simulink model "L4_SIM"  (R2018a)
settings: Solver=ode1  StartTime=0.0  StopTime=60  FixedStep=GLB_FIXED_STEP_SIZE_CPV  RelTol=1e-3  EnableMultiTasking=on
undefined symbols (not defined in the file or in its folder): Cf, Chassis, Cr, CYCLE_ACC1_2A__AdaptiveCruiseCtrlMode, CYCLE_ACC1_2A__AdaptiveCruiseCtrlSetSpeed, CYCLE_CCVS1_00__CruiseCtrlSetSpeed, CYCLE_CCVS1_00__WheelBasedVehicleSpeed, CYCLE_EEC1_00__EngSpeed, CYCLE_ETC1_00__TransDrivelineEngaged, CYCLE_ETC2_00__TransActualGearRatio, CYCLE_ETC7_03__TransMode1Indicator, CYCLE_GPS_Latitude, CYCLE_GPS_Longitude, CYCLE_LFE1_00__EngFuelRate, CYCLE_Net_Engine_Percent_Torque, CYCLE_SSI2_03__PitchAngleExRange, CYCLE_TIME, CYCLE_UTM_Origin_X, CYCLE_UTM_Origin_Y, CYCLE_Vehicle_Distance, DiscIntNeverNeededParam, ENUM_J1939_PCC_STATE_T, ENUM_J1939_SWITCH_T, ENUM_STEERING_WHEEL_ANGLE_SENSOR_TYPE_T, GLB_FIXED_STEP_SIZE_CPV, GLB_TRANS_LOSS_TRQ_GEAR_STEP_MPV, GLB_TRANS_LOSS_TRQ_SPD_STEP_MPV, GLB_TRANS_LOSS_TRQ_TABLE_DATA_MPV, GLB_TRANS_LOSS_TRQ_TRQ_STEP_MPV, GLB_VEHICLE_CONFIG_ACCEL_PED_GATEWAY_APV, heading_0, Iz, L4_Controller, lf, lr, position_0, ptc_matlab_lib, STEERCTRL_10ms, SUB_ECU_L4_MABX, SUB_L4_Task_10ms, SUB_L4_Task_10ms_SUB_STEERCTRL, SUB_PLANT_Chassis, Task_10ms, Vx_0
libraries: EmE_MBD_Blockset x81, PTC_MBDS_LIB x71, simulink x38, simulink_extras x1, SUB_L4_Task_10000ms x1, SUB_L4_Task_1000ms x1, SUB_L4_Task_100ms x1, SUB_L4_Task_10ms_SUB_APTC x1, SUB_L4_Task_10ms_SUB_BRKPEDARB x1, SUB_L4_Task_10ms_SUB_FAULT_MANAGER x1, SUB_L4_Task_10ms_SUB_STATE_CONTROL x1, simulink_need_slupdate x1
(part 3 of 6)

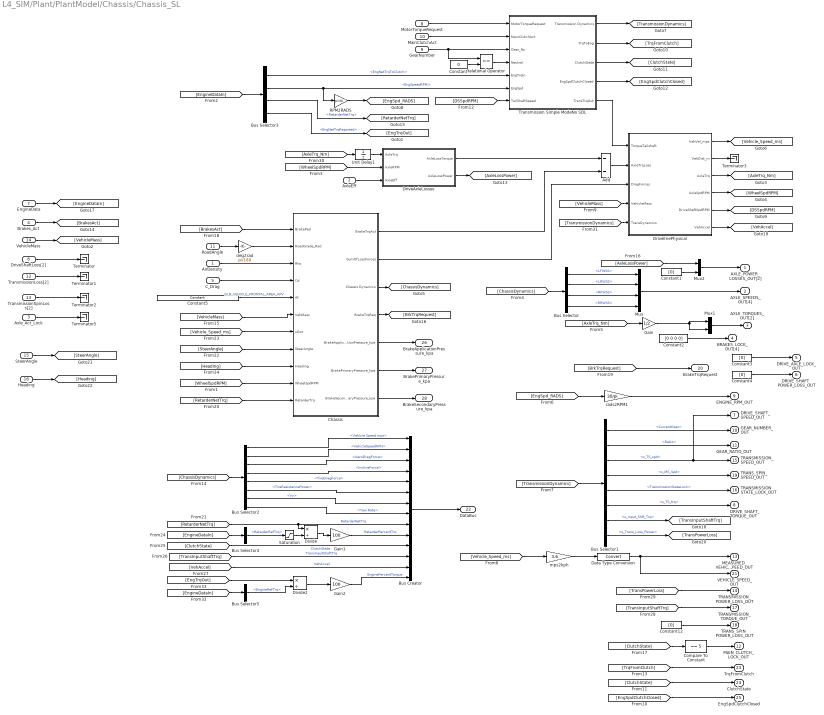
== system L4_SIM/Plant/PlantModel/Chassis/Chassis_SL ==
  AirDensity : Inport
  AxleEff : Inport  Port=2
  Axle_Act_Lock : Inport  Port=3
  Brakes_Act : Inport  Port=4
  C_Drag : Inport  Port=5
  DriveShaftLoss[2] : Inport  Port=6
  EngineData : Inport  Port=7
  MotorTorqueRequest : Inport  Port=8
  GearNumber : Inport  Port=9
  MainClutchAct : Inport  Port=10
  RoadAngle : Inport  Port=11
  TransmissionLoss[2] : Inport  Port=12
  TransmissionSpinLoss[2] : Inport  Port=13
  VehicleMass : Inport  Port=14
  SteerAngle : Inport  Port=15
  Heading : Inport  Port=16
  Add : Sum  Inputs=--
  Bus Creator : BusCreator  Inputs=14
  Bus Selector : BusSelector  OutputSignals=Wheel Speed Sensors.LFWSS,Wheel Speed Sensors.LRWSS,Wheel Speed Sensors.RFWSS,Wheel Speed Sensors.RRWSS
  Bus Selector1 : BusSelector  OutputSignals=Gears_bus.CurrentGear,Gears_bus.Ratio,Gears_bus.s_TS_spd,Gears_bus.s_MS_Spd,MainClutch_bus.TransmissionStateLock,Gears_bus.s_TS_trq,s_Input_Shft_Trq,Gears_bus.s_Trans_Loss_Power
  Bus Selector2 : BusSelector  OutputSignals=Vehicle Speed mps,VehicleSpeedKPH,LongitudnalDynamics.AeroDragForce,LongitudnalDynamics.InclineForce,LongitudnalDynamics.TireDragForce,TireResistancePower,LateralDynamics.Vy,LateralDynamics.Yaw Rate
  Bus Selector3 : BusSelector  OutputSignals=EngNetTrqToClutch,EngSpeedRPM,RetarderNetTrq,EngNetTrqReported
  Bus Selector4 : BusSelector  OutputSignals=RetarderRefTrq
  Bus Selector5 : BusSelector  OutputSignals=EngineRefTrq
  Chassis : Subsystem
  Compare To Constant : simulink/Logic and Bit Operations/Compare To Constant  relop===  const=5  OutDataTypeStr=boolean
  Constant : Constant  Value=0
  Constant{1,3..4,12} (4 alike) : Constant  Value=[0]
  Constant2 : Constant  Value=[0 0 0 0]
  Constant5 : PTC_MBDS_LIB/Extras/Sources/Constant  Value2=GLB_VEHICLE_FRONTAL_AREA_APV  PTC_MBDS_BlockVersion=5.41  PTC_BlockType=PTC_MBDS_Constant
      settings: SourceProductName=PACCAR Technical Center MBDS Library
      settings: AttributesFormatString=|
      | Value: 10.38
      | Unit: 'm^2'
  Data Type Conversion : DataTypeConversion  SaturateOnIntegerOverflow=on
  Divide : Product  Inputs=*/
  Divide2 : Product  Inputs=*/
  DriveAxleLosses : Subsystem
  DrivelInePhysical : Subsystem
  Gain : Gain  Gain=1/2
  Gain1 : Gain  Gain=100
  Gain2 : Gain  Gain=100
  Mux : Mux
  Mux1 : Mux  Inputs=2
  Mux2 : Mux  Inputs=2
  RPM2RADS : Gain  Gain=pi/30
  Relational Operator : RelationalOperator  Operator===  OutDataTypeStr=boolean  RndMeth=Nearest
  Saturation : Saturate  UpperLimit=inf  LowerLimit=1
  Terminator{,1..3,5} (5 alike) : Terminator
      Terminator3 settings: InitFcn=|
      | try
      |    MBDS_BlockCallback('Update', gcb);
      | end
  Transmission Simple ModeNo SDL : Subsystem
  Unit Delay1 : UnitDelay  SampleTime=-1
  deg2rad : Gain  Gain=pi/180
  mps2kph : Gain  Gain=3.6
  rads2RPM1 : Gain  Gain=30/pi
  AXLE_POWER_LOSSES_OUT[2] : Outport
  AXLE_SPEEDS_OUT[4] : Outport  Port=2
  AXLE_TORQUES_OUT[2] : Outport  Port=3
  BRAKES_LOCK_OUT[4] : Outport  Port=4
  DRIVE_AXLE_LOCK_OUT : Outport  Port=5
  DRIVE_SHAFT_POWER_LOSS_OUT : Outport  Port=6
  DRIVE_SHAFT_SPEED_OUT : Outport  Port=7
  DRIVE_SHAFT_TORQUE_OUT : Outport  Port=8
  ENGINE_RPM_OUT : Outport  Port=9
  GEAR_NUMBER_OUT : Outport  Port=10
  GEAR_RATIO_OUT : Outport  Port=11
  MAIN_CLUTCH_LOCK_OUT : Outport  Port=12
  MEASURED_VEHICLE_SPEED_OUT : Outport  Port=13
  TRANSMISSION_POWER_LOSS_OUT : Outport  Port=14
  TRANSMISSION_SPEED_OUT : Outport  Port=15
  TRANSMISSION_STATE_LOCK_OUT : Outport  Port=16
  TRANSMISSION_TORQUE_OUT : Outport  Port=17
  TRANS_SPIN_POWER_LOSS_OUT : Outport  Port=18
  TRANS_SPIN_SPEED_OUT : Outport  Port=19
  BrakeTrqRequest : Outport  Port=20
  VEHICLE_SPEED_OUT : Outport  Port=21
  DataBus : Outport  Port=22
  TrqFromClutch : Outport  Port=23
  ClutchState : Outport  Port=24
  EngSpdClutchClosed : Outport  Port=25
  BrakeApplicationPressure_kpa : Outport  Port=26
  BrakePrimaryPressure_kpa : Outport  Port=27
  BrakeSecondaryPressure_kpa : Outport  Port=28
  wires:
  DrivelInePhysical/1(VehVel_mps) -> [Vehicle_Speed_ms]
  Heading/1 -> [Heading]
  [Heading] -> Chassis/9(Heading)
  Bus Selector2/8 -> Bus Creator/8  "<Yaw Rate>"
  Bus Selector2/7 -> Bus Creator/7  "<Vy>"
  [SteerAngle] -> Chassis/8(SteerAngle)
  SteerAngle/1 -> [SteerAngle]
  Chassis/7(BrakeSecondaryPressure_kpa) -> BrakeSecondaryPressure_kpa/1
  Chassis/6(BrakePrimaryPressure_kpa) -> BrakePrimaryPressure_kpa/1
  Chassis/5(BrakeApplicationPressure_kpa) -> BrakeApplicationPressure_kpa/1
  Gain2/1 -> Bus Creator/14  "EnginePercentTorque"
  Divide2/1 -> Gain2/1
  [EngTrqOut] -> Divide2/1
  Bus Selector5/1 -> Divide2/2  "<EngineRefTrq>"
  [EngineDataIn] -> Bus Selector5/1
  Bus Selector/4 -> Mux/4  "<RRWSS>"
  Bus Selector/3 -> Mux/3  "<RFWSS>"
  Bus Selector/2 -> Mux/2  "<LRWSS>"
  Bus Selector/1 -> Mux/1  "<LFWSS>"
  Data Type Conversion/1 -> MEASURED_VEHICLE_SPEED_OUT/1, VEHICLE_SPEED_OUT/1
  Unit Delay1/1 -> DriveAxleLosses/1(AxleTrq)
  [TransmissionDynamics] -> DrivelInePhysical/5(TransDynamics)
  Bus Selector1/8 -> [TransPowerLoss]  "<s_Trans_Loss_Power>"
  Bus Selector2/5 -> Bus Creator/5  "<TireDragForce>"
  Saturation/1 -> Divide/2
  [VehAccel] -> Bus Creator/13  "VehAccel"
  DrivelInePhysical/6(VehAccel) -> [VehAccel]
  [TransInputShaftTrq] -> Bus Creator/12  "TransInputShaftTrq"
  Bus Selector1/7 -> [TransInputShaftTrq]  "<s_Input_Shft_Trq>"
  [ClutchState] -> Bus Creator/11  "ClutchState"
  Gain1/1 -> Bus Creator/10  "RetarderPercentTrq"
  Divide/1 -> Gain1/1
  Bus Selector4/1 -> Saturation/1  "<RetarderRefTrq>"
  [EngineDataIn] -> Bus Selector4/1
  EngineData/1 -> [EngineDataIn]
  Bus Selector2/6 -> Bus Creator/6  "<TireResistancePower>"
  Bus Selector2/4 -> Bus Creator/4  "<InclineForce>"
  Bus Selector2/3 -> Bus Creator/3  "<AeroDragForce>"
  Bus Selector2/2 -> Bus Creator/2  "<VehicleSpeedKPH>"
  Bus Selector2/1 -> Bus Creator/1  "<Vehicle Speed mps>"
  [RetarderNetTrq] -> Divide/1, Bus Creator/9  "RetarderNetTrq"
  Bus Creator/1 -> DataBus/1
  [RetarderNetTrq] -> Chassis/11(RetarderTrq)
  Chassis/4(BrakeTrqReq) -> [BrkTrqRequest]
  Bus Selector3/4 -> [EngTrqOut]  "<EngNetTrqReported>"
  Brakes_Act/1 -> [BrakesAct]
  [ClutchState] -> Compare To Constant/1
  Constant1/1 -> Mux2/2
  [AxleLossPower] -> Mux2/1
  DriveAxleLosses/2(AxleLossPower) -> [AxleLossPower]
  [VehicleMass] -> Chassis/6(VehMass)
  [ChassisDynamics] -> Bus Selector2/1
  RPM2RADS/1 -> [EngSpd_RADS]
  Transmission Simple ModeNo SDL/5(TransTrqOut) -> DrivelInePhysical/1(TorqueTailshaft)
  [EngSpdClutchClosed] -> EngSpdClutchClosed/1
  Transmission Simple ModeNo SDL/4(EngSpdClutchClosed) -> [EngSpdClutchClosed]
  Bus Selector3/1 -> Transmission Simple ModeNo SDL/5(EngTrqIn)  "<EngNetTrqToClutch>"
  [TrqFromClutch] -> TrqFromClutch/1
  [ClutchState] -> ClutchState/1
  Transmission Simple ModeNo SDL/3(ClutchState) -> [ClutchState]
  Transmission Simple ModeNo SDL/2(TrqToEng) -> [TrqFromClutch]
  [DSSpdRPM] -> Transmission Simple ModeNo SDL/7(TailShaftSpeed)
  DrivelInePhysical/5(DriveShaftSpdRPM) -> [DSSpdRPM]
  [VehicleMass] -> DrivelInePhysical/4(VehicleMass)
  VehicleMass/1 -> [VehicleMass]
  [WheelSpdRPM] -> Chassis/10(WheelSpdRPM)
  DrivelInePhysical/4(AxleSpdRPM) -> [WheelSpdRPM]
  Bus Selector1/3 -> DRIVE_SHAFT_SPEED_OUT/1, TRANSMISSION_SPEED_OUT/1  "<s_TS_spd>"
  [BrkTrqRequest] -> BrakeTrqRequest/1
  Bus Selector1/4 -> TRANS_SPIN_SPEED_OUT/1  "<s_MS_Spd>"
  Constant12/1 -> TRANS_SPIN_POWER_LOSS_OUT/1
  [TransInputShaftTrq] -> TRANSMISSION_TORQUE_OUT/1
  Bus Selector1/5 -> TRANSMISSION_STATE_LOCK_OUT/1  "<TransmissionStateLock>"
  [TransPowerLoss] -> TRANSMISSION_POWER_LOSS_OUT/1
  mps2kph/1 -> Data Type Conversion/1
  [Vehicle_Speed_ms] -> mps2kph/1
  Compare To Constant/1 -> MAIN_CLUTCH_LOCK_OUT/1
  Bus Selector1/2 -> GEAR_RATIO_OUT/1  "<Ratio>"
  Bus Selector1/1 -> GEAR_NUMBER_OUT/1  "<CurrentGear>"
  [TransmissionDynamics] -> Bus Selector1/1
  rads2RPM1/1 -> ENGINE_RPM_OUT/1
  [EngSpd_RADS] -> rads2RPM1/1
  Gain/1 -> Mux1/1, Mux1/2
  [AxleTrq_Nm] -> Gain/1
  Bus Selector1/6 -> DRIVE_SHAFT_TORQUE_OUT/1  "<s_TS_trq>"
  Constant4/1 -> DRIVE_SHAFT_POWER_LOSS_OUT/1
  Constant3/1 -> DRIVE_AXLE_LOCK_OUT/1
  Mux1/1 -> AXLE_TORQUES_OUT[2]/1
  Mux/1 -> AXLE_SPEEDS_OUT[4]/1
  Constant2/1 -> BRAKES_LOCK_OUT[4]/1
  Mux2/1 -> AXLE_POWER_LOSSES_OUT[2]/1
  [ChassisDynamics] -> Bus Selector/1
  Transmission Simple ModeNo SDL/1(Transmission Dynamics) -> [TransmissionDynamics]
  Chassis/3(Chassis Dynamics) -> [ChassisDynamics]
  Axle_Act_Lock/1 -> Terminator5/1
  TransmissionSpinLoss[2]/1 -> Terminator2/1
  TransmissionLoss[2]/1 -> Terminator1/1
  DriveShaftLoss[2]/1 -> Terminator/1
  [WheelSpdRPM] -> DriveAxleLosses/2(AxleRPM)
  AxleEff/1 -> DriveAxleLosses/3(AxleEff)
  [AxleTrq_Nm] -> Unit Delay1/1
  DrivelInePhysical/3(AxleTrq) -> [AxleTrq_Nm]
  Add/1 -> DrivelInePhysical/2(AxleTrqLoss)
  Chassis/1(BrakeTrqAct) -> Add/2
  DriveAxleLosses/1(AxleLossTorque) -> Add/1
  DrivelInePhysical/2(VehDist_m) -> Terminator3/1
  [Vehicle_Speed_ms] -> Chassis/7(xDot)
  [BrakesAct] -> Chassis/1(BrakePed)
  Chassis/2(SumOfLossForces) -> DrivelInePhysical/3(DragForces)
  Constant/1 -> Relational Operator/2
  Relational Operator/1 -> Transmission Simple ModeNo SDL/4(Neutral)
  GearNumber/1 -> Transmission Simple ModeNo SDL/3(Gear_No), Relational Operator/1
  MainClutchAct/1 -> Transmission Simple ModeNo SDL/2(MainClutchAct)
  deg2rad/1 -> Chassis/2(RoadGrade_Rad)
  RoadAngle/1 -> deg2rad/1
  Constant5/1 -> Chassis/5(Af)  "GLB_VEHICLE_FRONTAL_AREA_APV"
  C_Drag/1 -> Chassis/4(Cd)
  AirDensity/1 -> Chassis/3(Rho)
  [EngineDataIn] -> Bus Selector3/1
  Bus Selector3/2 -> RPM2RADS/1, Transmission Simple ModeNo SDL/6(EngSpd)  "<EngSpeedRPM>"
  Bus Selector3/3 -> [RetarderNetTrq]  "<RetarderNetTrq>"
  MotorTorqueRequest/1 -> Transmission Simple ModeNo SDL/1(MotorTorqueRequest)

== system L4_SIM/Controllers/Operator/Subsystem/SpdControlBrake/SpdControlBrake ==
  VehSpdTarget : Inport
  VehSpdAct : Inport  Port=2
  Kp : Inport  Port=3
  Ti : Inport  Port=4
  Td : Inport  Port=5
  Reset : Inport  Port=6
  Constant : Constant  Value=0
  Constant1 : Constant  Value=0
  Constant2 : Constant  Value=-1
  Constant3 : Constant
  Constant4 : PTC_MBDS_LIB/Extras/Sources/Constant  Value2=GLB_FIXED_STEP_SIZE_CPV  PTC_MBDS_BlockVersion=5.41  PTC_BlockType=PTC_MBDS_Constant
      settings: SourceProductName=PACCAR Technical Center MBDS Library
      settings: AttributesFormatString=|
      | Value: 0.01
      | Unit: 's'
  Constant7 : Constant
  Constant8 : Constant  Value=0
  Gain : Gain  Gain=-1
  Mux : Mux
  PID : Subsystem
  Relational Operator : RelationalOperator  OutDataTypeStr=boolean  RndMeth=Nearest
  Relational Operator1 : RelationalOperator  Operator=<=  OutDataTypeStr=boolean  RndMeth=Nearest
  Saturation Dynamic : simulink/Discontinuities/Saturation Dynamic  RequirementInfo={} %GIDa_73e9c469_c4a7_47ae_bea8_3c2217de47e7  OutMin=[]  OutMax=[]  OutDataTypeStr=Inherit: Same as second input  OutDataType=sfix(16)  OutScaling=2^-10  DoSatur=off
  Switch : Switch  Criteria=u2 ~= 0
  Switch1 : Switch  Criteria=u2 ~= 0
  Terminator : Terminator
  Unit Delay : UnitDelay  SampleTime=-1
  BrakeComGov(0-1) : Outport
  wires:
  Reset/1 -> PID/2(Reset_Integral)
  Saturation Dynamic/1 -> BrakeComGov(0-1)/1
  Gain/1 -> Saturation Dynamic/2, Unit Delay/1
  Td/1 -> PID/7(Td)
  Unit Delay/1 -> Relational Operator1/1, Relational Operator/1
  Constant8/1 -> Saturation Dynamic/3, Relational Operator1/2
  Constant7/1 -> Saturation Dynamic/1, Relational Operator/2
  Relational Operator/1 -> Switch/2
  Constant3/1 -> Switch/1
  Switch1/1 -> Switch/3
  Constant2/1 -> Switch1/1
  Constant/1 -> Switch1/3
  Relational Operator1/1 -> Switch1/2
  Switch/1 -> PID/9(Sat_state)
  PID/4(D_Out1) -> Mux/4
  PID/3(I_Out) -> Mux/3
  PID/2(P_Out) -> Mux/2
  Mux/1 -> Terminator/1
  Constant1/1 -> PID/1(Init)
  Kp/1 -> PID/5(K)
  Ti/1 -> PID/6(Ti)
  Constant4/1 -> PID/8(Ts)  "GLB_FIXED_STEP_SIZE_CPV"
  VehSpdTarget/1 -> PID/3(SP)
  VehSpdAct/1 -> PID/4(FB)
  PID/1(Out1) -> Gain/1, Mux/1

== system L4_SIM/Controllers/Operator/Subsystem/SpdControlTraction/SpdControlTraction ==
  VehSpdTarget : Inport
  VehSpdAct : Inport  Port=2
  Kp : Inport  Port=3
  Ti : Inport  Port=4
  Td : Inport  Port=5
  Reset : Inport  Port=6
  Constant : Constant  Value=0
  Constant1 : Constant  Value=0
  Constant2 : Constant  Value=-1
  Constant3 : Constant
  Constant4 : PTC_MBDS_LIB/Extras/Sources/Constant  Value2=GLB_FIXED_STEP_SIZE_CPV  PTC_MBDS_BlockVersion=5.41  PTC_BlockType=PTC_MBDS_Constant
      settings: SourceProductName=PACCAR Technical Center MBDS Library
      settings: AttributesFormatString=|
      | Value: 0.01
      | Unit: 's'
  Constant7 : Constant
  Constant8 : Constant  Value=0
  Mux : Mux
  PID : Subsystem
  Relational Operator : RelationalOperator  OutDataTypeStr=boolean  RndMeth=Nearest
  Relational Operator1 : RelationalOperator  Operator=<=  OutDataTypeStr=boolean  RndMeth=Nearest
  Saturation : Saturate  UpperLimit=1  LowerLimit=0
  Switch : Switch  Criteria=u2 ~= 0
  Switch1 : Switch  Criteria=u2 ~= 0
  Terminator : Terminator
  Unit Delay : UnitDelay  SampleTime=-1
  PedalComGov(0-1) : Outport
  wires:
  Switch/1 -> PID/9(Sat_state)
  Unit Delay/1 -> Relational Operator1/1, Relational Operator/1
  Constant8/1 -> Relational Operator1/2
  Constant7/1 -> Relational Operator/2
  Relational Operator/1 -> Switch/2
  Constant3/1 -> Switch/1
  Switch1/1 -> Switch/3
  Constant2/1 -> Switch1/1
  Constant/1 -> Switch1/3
  Relational Operator1/1 -> Switch1/2
  PID/4(D_Out1) -> Mux/4
  PID/3(I_Out) -> Mux/3
  PID/2(P_Out) -> Mux/2
  Mux/1 -> Terminator/1
  Constant4/1 -> PID/8(Ts)  "GLB_FIXED_STEP_SIZE_CPV"
  PID/1(Out1) -> Unit Delay/1, Saturation/1, Mux/1
  Saturation/1 -> PedalComGov(0-1)/1
  VehSpdTarget/1 -> PID/3(SP)
  VehSpdAct/1 -> PID/4(FB)
  Kp/1 -> PID/5(K)
  Ti/1 -> PID/6(Ti)
  Td/1 -> PID/7(Td)
  Constant1/1 -> PID/1(Init)
  Reset/1 -> PID/2(Reset_Integral)

== system L4_SIM/Controllers/Virtual_Controllers/Interface_Abstraction/CAN/ACC1 ==
  SPN1586_SpeedOfForwardVehicle : Inport
  SPN1587_DistanceToForwardVehicle : Inport  Port=2
  SPN1588_AdaptiveCruiseControlSetSpeed : Inport  Port=3
  SPN1590_AdaptiveCruiseControlMode : Inport  Port=4
  SPN1589_AdaptiveCruiseControlSetDistMode : Inport  Port=5
  SPN1591_RoadCurvature : Inport  Port=6
  SPN1798_ACC_TargetDetected : Inport  Port=7
  SPN1797_ACC_SystemShutoffWarning : Inport  Port=8
  SPN1796_ACC_DistanceAlertSignal : Inport  Port=9
  SPN5022_ForwardCollisionWarning : Inport  Port=10
  Bus Creator2 : BusCreator  Inputs=10
  ACC1 : Outport
  wires:
  SPN1586_SpeedOfForwardVehicle/1 -> Bus Creator2/1  "SPN1586_SpeedOfForwardVehicle"
  Bus Creator2/1 -> ACC1/1  "ACC1"
  SPN1587_DistanceToForwardVehicle/1 -> Bus Creator2/2  "SPN1587_DistanceToForwardVehicle"
  SPN1588_AdaptiveCruiseControlSetSpeed/1 -> Bus Creator2/3  "SPN1588_AdaptiveCruiseControlSetSpeed"
  SPN1590_AdaptiveCruiseControlMode/1 -> Bus Creator2/4  "SPN1590_AdaptiveCruiseControlMode"
  SPN1797_ACC_SystemShutoffWarning/1 -> Bus Creator2/8  "SPN1797_ACC_SystemShutoffWarning"
  SPN1798_ACC_TargetDetected/1 -> Bus Creator2/7  "SPN1798_ACC_TargetDetected"
  SPN1591_RoadCurvature/1 -> Bus Creator2/6  "SPN1591_RoadCurvature"
  SPN1589_AdaptiveCruiseControlSetDistMode/1 -> Bus Creator2/5  "SPN1589_AdaptiveCruiseControlSetDistMode"
  SPN1796_ACC_DistanceAlertSignal/1 -> Bus Creator2/9  "SPN1796_ACC_DistanceAlertSignal"
  SPN5022_ForwardCollisionWarning/1 -> Bus Creator2/10  "SPN5022_ForwardCollisionWarning"

== system L4_SIM/Controllers/Virtual_Controllers/Interface_Abstraction/CAN/AMB ==
  SPN108_BarometricPressure : Inport
  SPN171_AmbientAirTemperature : Inport  Port=2
  SPN170_CabInteriorTemperature : Inport  Port=3
  Bus Creator2 : BusCreator  Inputs=3
  AMB : Outport
  wires:
  Bus Creator2/1 -> AMB/1
  SPN108_BarometricPressure/1 -> Bus Creator2/1  "SPN108_BarometricPressure"
  SPN171_AmbientAirTemperature/1 -> Bus Creator2/2  "SPN171_AmbientAirTemperature"
  SPN170_CabInteriorTemperature/1 -> Bus Creator2/3  "SPN170_CabInteriorTemperature"

== system L4_SIM/Controllers/Virtual_Controllers/Interface_Abstraction/CAN/BrakeSwitch ==
  In : Inport
  Compare To Constant : simulink/Logic and Bit Operations/Compare To Constant  relop=>=  const=0.05  OutDataTypeStr=boolean
  Out : Outport
  wires:
  In/1 -> Compare To Constant/1
  Compare To Constant/1 -> Out/1

== system L4_SIM/Controllers/Virtual_Controllers/Interface_Abstraction/CAN/CC ==
  CCSetSpd : Inport
  Constant : Constant  Value=20
  Constant1 : Constant
  Constant2 : Constant  Value=0
  Relational Operator : RelationalOperator  Operator=>  OutDataTypeStr=boolean  RndMeth=Nearest
  Switch : Switch  Criteria=u2 ~= 0
  CruiseActive : Outport
  CruiseState : Outport  Port=2
  wires:
  Relational Operator/1 -> Switch/2, CruiseActive/1
  Constant/1 -> Relational Operator/2
  CCSetSpd/1 -> Relational Operator/1
  Switch/1 -> CruiseState/1
  Constant1/1 -> Switch/1
  Constant2/1 -> Switch/3

== system L4_SIM/Controllers/Virtual_Controllers/Interface_Abstraction/CAN/CCVS1 ==
  SPN84_WheelBasedVehicleSpeed : Inport
  SPN597_BrakeSwitch : Inport  Port=2
  SPN86_CruiseControlSetSpeed : Inport  Port=3
  SPN595_CruiseControlActive : Inport  Port=4
  SPN527_CruiseControlState : Inport  Port=5
  Bus Creator2 : BusCreator  Inputs=5
  CCVS1 : Outport
  wires:
  SPN84_WheelBasedVehicleSpeed/1 -> Bus Creator2/1
  Bus Creator2/1 -> CCVS1/1
  SPN597_BrakeSwitch/1 -> Bus Creator2/2
  SPN86_CruiseControlSetSpeed/1 -> Bus Creator2/3
  SPN595_CruiseControlActive/1 -> Bus Creator2/4
  SPN527_CruiseControlState/1 -> Bus Creator2/5

== system L4_SIM/Controllers/Virtual_Controllers/Interface_Abstraction/CAN/CCVS3 ==
  SPN7319_CruiseControlSpeed : Inport
  Bus Creator2 : BusCreator  Inputs=1
  CCVS3 : Outport
  wires:
  Bus Creator2/1 -> CCVS3/1
  SPN7319_CruiseControlSpeed/1 -> Bus Creator2/1

== system L4_SIM/Controllers/Virtual_Controllers/Interface_Abstraction/CAN/CVW ==
  SPN1760_GrossCombinationVehicleWeight : Inport
  Bus Creator2 : BusCreator  Inputs=1
  CVW : Outport
  wires:
  Bus Creator2/1 -> CVW/1
  SPN1760_GrossCombinationVehicleWeight/1 -> Bus Creator2/1

== system L4_SIM/Controllers/Virtual_Controllers/Interface_Abstraction/CAN/EBC1 ==
  SPN521_BrakePedalPosition : Inport
  Bus Creator2 : BusCreator  Inputs=2
  Constant : Constant  Value=0
  Relational Operator : RelationalOperator  Operator=>  OutDataTypeStr=boolean  RndMeth=Simplest
  EBC1 : Outport
  wires:
  SPN521_BrakePedalPosition/1 -> Relational Operator/1, Bus Creator2/1
  Bus Creator2/1 -> EBC1/1
  Constant/1 -> Relational Operator/2
  Relational Operator/1 -> Bus Creator2/2  "SPN1121_EBS_BrakeSwitch"

== system L4_SIM/Controllers/Virtual_Controllers/Interface_Abstraction/CAN/EBC2 ==
  SPN904_FrontAxleSpd : Inport  Unit=km/h
  Bus Creator2 : BusCreator  Inputs=1
  EBC2 : Outport
  wires:
  Bus Creator2/1 -> EBC2/1
  SPN904_FrontAxleSpd/1 -> Bus Creator2/1  "SPN904_FrontAxleSpd"

== system L4_SIM/Controllers/Virtual_Controllers/Interface_Abstraction/CAN/EC1 ==
  SPN544_EngineReferenceTrq : Inport
  Bus Creator2 : BusCreator  Inputs=1
  EC1 : Outport
  wires:
  SPN544_EngineReferenceTrq/1 -> Bus Creator2/1  "SPN544_EngineReferenceTrq"
  Bus Creator2/1 -> EC1/1

== system L4_SIM/Controllers/Virtual_Controllers/Interface_Abstraction/CAN/EEC1 ==
  SPN512_DriverDemandPercTorque : Inport
  SPN513_ActualEngPercTorque : Inport  Port=2
  SPN4154_ActualEngPercTorqueFractional : Inport  Port=3
  SPN190_EngineSpeed : Inport  Port=4
  Bus Creator : BusCreator  Inputs=4
  EEC1 : Outport
  wires:
  Bus Creator/1 -> EEC1/1
  SPN190_EngineSpeed/1 -> Bus Creator/4
  SPN4154_ActualEngPercTorqueFractional/1 -> Bus Creator/3
  SPN513_ActualEngPercTorque/1 -> Bus Creator/2
  SPN512_DriverDemandPercTorque/1 -> Bus Creator/1

== system L4_SIM/Controllers/Virtual_Controllers/Interface_Abstraction/CAN/EEC2 ==
  SPN91_AccelPedalPosition1 : Inport
  Bus Creator2 : BusCreator  Inputs=1
  EEC2 : Outport
  wires:
  Bus Creator2/1 -> EEC2/1
  SPN91_AccelPedalPosition1/1 -> Bus Creator2/1

== system L4_SIM/Controllers/Virtual_Controllers/Interface_Abstraction/CAN/EEC3 ==
  SPN514_NominalFrictionPercTorque : Inport
  SPN2978_EstimatedEngineParasiticLossesPercTrq : Inport  Port=2
  Bus Creator2 : BusCreator  Inputs=2
  EEC3 : Outport
  wires:
  Bus Creator2/1 -> EEC3/1
  SPN514_NominalFrictionPercTorque/1 -> Bus Creator2/1  "SPN514_NominalFrictionPercTorque"
  SPN2978_EstimatedEngineParasiticLossesPercTrq/1 -> Bus Creator2/2  "SPN2978_EstimatedEngineParasiticLossesPercTrq"

== system L4_SIM/Controllers/Virtual_Controllers/Interface_Abstraction/CAN/ERC1 ==
  SPN520_ActualRetarderPercentTorque : Inport
  SPN1715_DriverDemandRetarderPercentTorque : Inport  Port=2
  Bus Creator2 : BusCreator  Inputs=2
  ERC1 : Outport
  wires:
  SPN520_ActualRetarderPercentTorque/1 -> Bus Creator2/1
  Bus Creator2/1 -> ERC1/1
  SPN1715_DriverDemandRetarderPercentTorque/1 -> Bus Creator2/2

== system L4_SIM/Controllers/Virtual_Controllers/Interface_Abstraction/CAN/ETC1 ==
  SPN560_TransDrivelineEngaged : Inport
  Bus Creator2 : BusCreator  Inputs=1
  ETC1 : Outport
  wires:
  Bus Creator2/1 -> ETC1/1  "ETC1"
  SPN560_TransDrivelineEngaged/1 -> Bus Creator2/1

== system L4_SIM/Controllers/Virtual_Controllers/Interface_Abstraction/CAN/ETC2 ==
  SPN524_TransSelectedGear : Inport
  SPN526_TransActualGearRatio : Inport  Port=2
  SPN523_TransCurrentGear : Inport  Port=3
  Bus Creator1 : BusCreator  Inputs=3
  ETC2 : Outport
  wires:
  Bus Creator1/1 -> ETC2/1
  SPN526_TransActualGearRatio/1 -> Bus Creator1/2
  SPN523_TransCurrentGear/1 -> Bus Creator1/3
  SPN524_TransSelectedGear/1 -> Bus Creator1/1

== system L4_SIM/Controllers/Virtual_Controllers/Interface_Abstraction/CAN/GNSSSDOP ==
  SID : Inport
  SetMode : Inport  Port=2
  OpMode : Inport  Port=3
  HDOP : Inport  Port=4
  VDOP : Inport  Port=5
  TDOP : Inport  Port=6
  Bus Creator2 : BusCreator  Inputs=6
  GNSSDOP : Outport
  wires:
  Bus Creator2/1 -> GNSSDOP/1
  SID/1 -> Bus Creator2/1  "SID"
  SetMode/1 -> Bus Creator2/2  "SetMode"
  OpMode/1 -> Bus Creator2/3  "OpMode"
  HDOP/1 -> Bus Creator2/4  "HDOP"
  VDOP/1 -> Bus Creator2/5  "VDOP"
  TDOP/1 -> Bus Creator2/6  "TDOP"

== system L4_SIM/Controllers/Virtual_Controllers/Interface_Abstraction/CAN/HRW ==
  SPN1592_FrontAxleLeftWheelSpeed : Inport  Unit=km/h
  SPN1593_FrontAxleRightWheelSpeed : Inport  Port=2  Unit=km/h
  SPN1594_RearAxleLeftWheelSpeed : Inport  Port=3  Unit=km/h
  SPN1595_RearAxleRightWheelSpeed : Inport  Port=4  Unit=km/h
  Bus Creator2 : BusCreator  Inputs=4
  HRW_0B : Outport
  wires:
  SPN1592_FrontAxleLeftWheelSpeed/1 -> Bus Creator2/1  "SPN1592_FrontAxleLeftWheelSpeed"
  Bus Creator2/1 -> HRW_0B/1
  SPN1593_FrontAxleRightWheelSpeed/1 -> Bus Creator2/2  "SPN1593_FrontAxleRightWheelSpeed"
  SPN1594_RearAxleLeftWheelSpeed/1 -> Bus Creator2/3  "SPN1594_RearAxleLeftWheelSpeed"
  SPN1595_RearAxleRightWheelSpeed/1 -> Bus Creator2/4  "SPN1595_RearAxleRightWheelSpeed"

== system L4_SIM/Controllers/Virtual_Controllers/Interface_Abstraction/CAN/PCC1 ==
  SPN7316_PCCSetSpeedOffset : Inport
  SPN7317_PCCState : Inport  Port=2
  SPN7430_PCCDrivelineDisengageInhibit : Inport  Port=3
  Bus Creator2 : BusCreator  Inputs=3
  PCC1 : Outport
  wires:
  Bus Creator2/1 -> PCC1/1
  SPN7316_PCCSetSpeedOffset/1 -> Bus Creator2/1
  SPN7317_PCCState/1 -> Bus Creator2/2
  SPN7430_PCCDrivelineDisengageInhibit/1 -> Bus Creator2/3

== system L4_SIM/Controllers/Virtual_Controllers/Interface_Abstraction/CAN/PosRapidUpdate ==
  Latitude : Inport
  Longitude : Inport  Port=2
  Bus Creator2 : BusCreator  Inputs=2
  PosRapidUpdate : Outport
  wires:
  Longitude/1 -> Bus Creator2/2  "Longitude"
  Latitude/1 -> Bus Creator2/1  "Latitude"
  Bus Creator2/1 -> PosRapidUpdate/1

== system L4_SIM/Controllers/Virtual_Controllers/Interface_Abstraction/CAN/SSI2 ==
  SPN4976_PitchAngleExtendedRange : Inport
  Bus Creator2 : BusCreator  Inputs=1
  SSI2 : Outport
  wires:
  SPN4976_PitchAngleExtendedRange/1 -> Bus Creator2/1
  Bus Creator2/1 -> SSI2/1  "ETC1"

== system L4_SIM/Controllers/Virtual_Controllers/Interface_Abstraction/CAN/TransDrivelineEngaged ==
  In1 : Inport
  Constant : PTC_MBDS_LIB/Extras/Sources/Constant  Value2=ENUM_J1939_SWITCH_T.ON  PTC_MBDS_BlockVersion=5.41  PTC_BlockType=PTC_MBDS_Constant
      settings: SourceProductName=PACCAR Technical Center MBDS Library
  Constant1 : PTC_MBDS_LIB/Extras/Sources/Constant  Value2=ENUM_J1939_SWITCH_T.OFF  PTC_MBDS_BlockVersion=5.41  PTC_BlockType=PTC_MBDS_Constant
      settings: SourceProductName=PACCAR Technical Center MBDS Library
  Data Type Conversion : DataTypeConversion  SaturateOnIntegerOverflow=on
  If_Then_Else : PTC_MBDS_LIB/Extras/Signal Routing/If_Then_Else  PTC_MBDS_BlockVersion=5.41  PTC_BlockType=PTC_MBDS_If_Then_Else
      settings: SourceProductName=PACCAR Technical Center MBDS Library
  Out1 : Outport
  wires:
  In1/1 -> Data Type Conversion/1
  Constant/1 -> If_Then_Else/2
  Constant1/1 -> If_Then_Else/3
  If_Then_Else/1 -> Out1/1
  Data Type Conversion/1 -> If_Then_Else/1

== system L4_SIM/Controllers/Virtual_Controllers/Interface_Abstraction/CAN/VDC1 ==
  SPN1813_VDC_InformationSignal : Inport
  SPN1814_VDC_FullyOperational : Inport  Port=2
  SPN1815_VDC_BrakeLightRequest : Inport  Port=3
  SPN1816_ROP_EngineControlActive : Inport  Port=4
  SPN1818_ROP_BrakeControlActive : Inport  Port=5
  SPN1817_YC_EngineControlActive : Inport  Port=6
  SPN1819_YC_BrakeControlActive : Inport  Port=7
  SPN5624_TrailerVDC_Active : Inport  Port=8
  Bus Creator2 : BusCreator  Inputs=8
  VDC1 : Outport
  wires:
  SPN1816_ROP_EngineControlActive/1 -> Bus Creator2/4  "SPN1816_ROP_EngineControlActive"
  SPN1815_VDC_BrakeLightRequest/1 -> Bus Creator2/3  "SPN1815_VDC_BrakeLightRequest"
  SPN1813_VDC_InformationSignal/1 -> Bus Creator2/1  "SPN1813_VDC_InformationSignal"
  SPN1814_VDC_FullyOperational/1 -> Bus Creator2/2  "SPN1814_VDC_FullyOperational"
  Bus Creator2/1 -> VDC1/1
  SPN1818_ROP_BrakeControlActive/1 -> Bus Creator2/5  "SPN1818_ROP_BrakeControlActive"
  SPN1817_YC_EngineControlActive/1 -> Bus Creator2/6  "SPN1817_YC_EngineControlActive"
  SPN1819_YC_BrakeControlActive/1 -> Bus Creator2/7  "SPN1819_YC_BrakeControlActive"
  SPN5624_TrailerVDC_Active/1 -> Bus Creator2/8  "SPN5624_TrailerVDC_Active"

== system L4_SIM/Controllers/Virtual_Controllers/Interface_Abstraction/CAN/VDC2 ==
  SPN1807_SteeringWheelAngle : Inport
  SPN1808_YawRate : Inport  Port=2
  SPN1809_LateralAcceleration : Inport  Port=3
  SPN1810_LongitudinalAcceleration : Inport  Port=4
  SPN1811_SteeringWheelTurnCounter : Inport  Port=5
  SPN1812_SteeringWheelAngleSensorType : Inport  Port=6
  Bus Creator2 : BusCreator  Inputs=6
  VDC2 : Outport
  wires:
  Bus Creator2/1 -> VDC2/1
  SPN1808_YawRate/1 -> Bus Creator2/2  "SPN1808_YawRate"
  SPN1807_SteeringWheelAngle/1 -> Bus Creator2/1  "SPN1807_SteeringWheelAngle"
  SPN1809_LateralAcceleration/1 -> Bus Creator2/3  "SPN1809_LateralAcceleration"
  SPN1810_LongitudinalAcceleration/1 -> Bus Creator2/4  "SPN1810_LongitudinalAcceleration"
  SPN1811_SteeringWheelTurnCounter/1 -> Bus Creator2/5  "SPN1811_SteeringWheelTurnCounter"
  SPN1812_SteeringWheelAngleSensorType/1 -> Bus Creator2/6  "SPN1812_SteeringWheelAngleSensorType"

== system L4_SIM/Controllers/Virtual_Controllers/Interface_Abstraction/CAN/VDHR ==
  SPN917_TotalVehicleDistanceHiResolution : Inport
  Bus Creator2 : BusCreator  Inputs=1
  VDHR : Outport
  wires:
  SPN917_TotalVehicleDistanceHiResolution/1 -> Bus Creator2/1
  Bus Creator2/1 -> VDHR/1

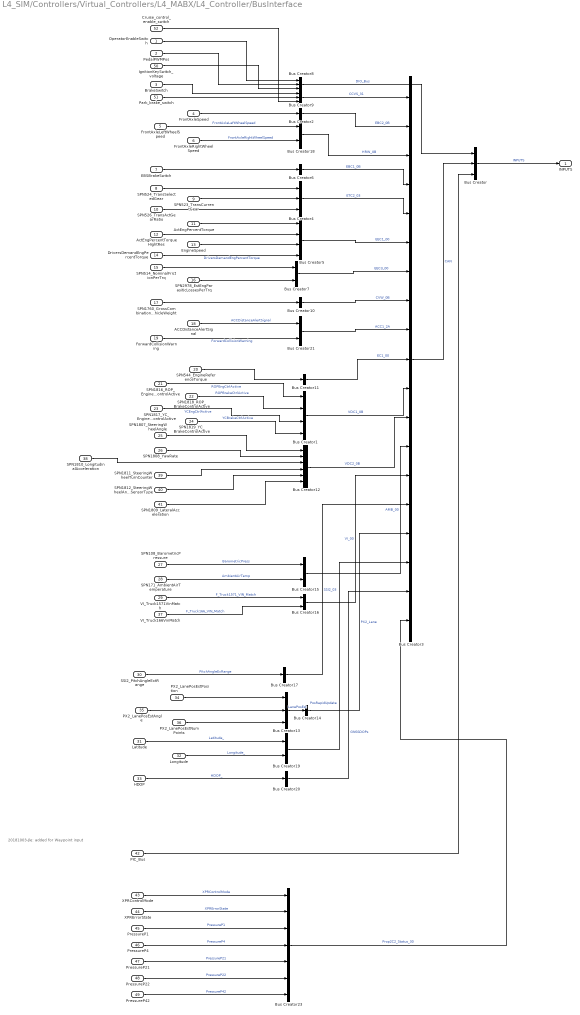
== system L4_SIM/Controllers/Virtual_Controllers/L4_MABX/L4_Controller/BusInterface ==
  note: 20181003-Jle: added for Waypoint input
  OperatorEnableSwitch : Inport
  PedalPWMPos : Inport  Port=2
  BrakeSwitch : Inport  Port=3
  FrontAxleSpeed : Inport  Port=4
  FrontAxleLeftWheelSpeed : Inport  Port=5
  FrontAxleRightWheelSpeed : Inport  Port=6
  EBSBrakeSwitch : Inport  Port=7
  SPN524_TransSelectedGear : Inport  Port=8
  SPN523_TransCurrentGear : Inport  Port=9
  SPN526_TransActGearRatio : Inport  Port=10
  ActEngPercentTorque : Inport  Port=11
  ActEngPercentTorqueHightRes : Inport  Port=12
  EngineSpeed : Inport  Port=13
  DriversDemandEngPercentTorque : Inport  Port=14
  SPN514_NominalFrictionPerTrq : Inport  Port=15
  SPN2978_EstEngParasiticLossesPerTrq : Inport  Port=16
  SPN1760_GrossCombinationVehicleWeight : Inport  Port=17
  ACCDistanceAlertSignal : Inport  Port=18
  ForwardCollisionWarning : Inport  Port=19
  SPN544_EngineReferenceTorque : Inport  Port=20
  SPN1816_ROP_EngineControlActive : Inport  Port=21
  SPN1818_ROP_BrakeControlActive : Inport  Port=22
  SPN1817_YC_EngineControlActive : Inport  Port=23
  SPN1819_YC_BrakeControlActive : Inport  Port=24
  SPN1807_SteeringWheelAngle : Inport  Port=25
  SPN1808_YawRate : Inport  Port=26
  SPN108_BarometricPressure : Inport  Port=27
  SPN171_AmbientAirTemperature : Inport  Port=28
  VI_Truck1571VinMatch : Inport  Port=29
  SSI2_PitchAngleExtRange : Inport  Port=30
  Latitude : Inport  Port=31
  Longitude : Inport  Port=32
  HDOP : Inport  Port=33
  PX2_LanePosEstPosition : Inport  Port=34
  PX2_LanePosEstAngle : Inport  Port=35
  PX2_LanePosEstNumPoints : Inport  Port=36
  VI_Truck166VinMatch : Inport  Port=37
  SPN1810_LongitudinalAcceleration : Inport  Port=38
  SPN1811_SteeringWheelTurnCounter : Inport  Port=39
  SPN1812_SteeringWheelAngleSensorType : Inport  Port=40
  SPN1809_LateralAcceleration : Inport  Port=41
  PIC_Bus : Inport  Port=42
  XPRControlMode : Inport  Port=43
  XPRErrorState : Inport  Port=44
  PressureP1 : Inport  Port=45
  PressureP4 : Inport  Port=46
  PressureP21 : Inport  Port=47
  PressureP22 : Inport  Port=48
  PressureP42 : Inport  Port=49
  IgnitionKeySwitch_voltage : Inport  Port=50
  Park_brake_switch : Inport  Port=51
  Cruise_control_enable_switch : Inport  Port=52
  Bus Creator{,4,8..9,13} (5 alike) : BusCreator  Inputs=3
  Bus Creator1 : BusCreator  Inputs=4
  Bus Creator{2,6,10..11,14,17,20} (7 alike) : BusCreator  Inputs=1
  Bus Creator12 : BusCreator  Inputs=6
  Bus Creator{7,15..16,18..19,21} (6 alike) : BusCreator  Inputs=2
  Bus Creator23 : BusCreator  Inputs=7
  Bus Creator3 : BusCreator  Inputs=19
  Bus Creator5 : BusCreator  Inputs=4
  INPUTS : Outport
  wires:
  Bus Creator23/1 -> Bus Creator3/19  "Prop2C2_Status_30"
  XPRControlMode/1 -> Bus Creator23/1  "XPRControlMode"
  PressureP21/1 -> Bus Creator23/5  "PressureP21"
  XPRErrorState/1 -> Bus Creator23/2  "XPRErrorState"
  PressureP42/1 -> Bus Creator23/7  "PressureP42"
  PressureP1/1 -> Bus Creator23/3  "PressureP1"
  PressureP22/1 -> Bus Creator23/6  "PressureP22"
  PressureP4/1 -> Bus Creator23/4  "PressureP4"
  SPN1809_LateralAcceleration/1 -> Bus Creator12/6
  SPN1812_SteeringWheelAngleSensorType/1 -> Bus Creator12/5
  SPN1811_SteeringWheelTurnCounter/1 -> Bus Creator12/4
  SPN1810_LongitudinalAcceleration/1 -> Bus Creator12/3
  VI_Truck166VinMatch/1 -> Bus Creator16/2  "F_Truck166_VIN_Match"
  Bus Creator1/1 -> Bus Creator3/11  "VDC1_0B"
  SPN1819_YC_BrakeControlActive/1 -> Bus Creator1/4  "YCBrakeCtrlActive"
  SPN1817_YC_EngineControlActive/1 -> Bus Creator1/3  "YCEngCtrlActive"
  SPN1818_ROP_BrakeControlActive/1 -> Bus Creator1/2  "ROPBrakeCtrlActive"
  SPN1816_ROP_EngineControlActive/1 -> Bus Creator1/1  "ROPEngCtrlActive"
  SPN1808_YawRate/1 -> Bus Creator12/2
  Bus Creator/1 -> INPUTS/1  "INPUTS"
  EngineSpeed/1 -> Bus Creator5/3
  PX2_LanePosEstPosition/1 -> Bus Creator13/1
  FrontAxleSpeed/1 -> Bus Creator2/1
  SPN1807_SteeringWheelAngle/1 -> Bus Creator12/1
  Bus Creator14/1 -> Bus Creator3/16  "PX2_Lane"
  SPN526_TransActGearRatio/1 -> Bus Creator4/3
  SPN544_EngineReferenceTorque/1 -> Bus Creator11/1
  Bus Creator12/1 -> Bus Creator3/12  "VDC2_0B"
  Bus Creator6/1 -> Bus Creator3/4  "EBC1_0B"
  Bus Creator4/1 -> Bus Creator3/5  "ETC2_03"
  SPN2978_EstEngParasiticLossesPerTrq/1 -> Bus Creator7/2
  SPN514_NominalFrictionPerTrq/1 -> Bus Creator7/1
  SPN524_TransSelectedGear/1 -> Bus Creator4/1
  Bus Creator2/1 -> Bus Creator3/2  "EBC2_0B"
  SPN523_TransCurrentGear/1 -> Bus Creator4/2
  Bus Creator9/1 -> Bus Creator3/1  "CCVS_31"
  Bus Creator10/1 -> Bus Creator3/8  "CVW_0B"
  PX2_LanePosEstAngle/1 -> Bus Creator13/2
  SPN1760_GrossCombinationVehicleWeight/1 -> Bus Creator10/1
  Bus Creator7/1 -> Bus Creator3/7  "EEC3_00"
  ActEngPercentTorqueHightRes/1 -> Bus Creator5/2
  Bus Creator11/1 -> Bus Creator3/10  "EC1_00"
  EBSBrakeSwitch/1 -> Bus Creator6/1
  BrakeSwitch/1 -> Bus Creator9/1
  Bus Creator3/1 -> Bus Creator/2  "CAN"
  ActEngPercentTorque/1 -> Bus Creator5/1
  OperatorEnableSwitch/1 -> Bus Creator8/1
  Bus Creator5/1 -> Bus Creator3/6  "EEC1_00"
  PX2_LanePosEstNumPoints/1 -> Bus Creator13/3
  Bus Creator8/1 -> Bus Creator/1  "DIO_Bus"
  Bus Creator13/1 -> Bus Creator14/1  "LanePosEst"
  SPN108_BarometricPressure/1 -> Bus Creator15/1  "BarometricPress"
  SPN171_AmbientAirTemperature/1 -> Bus Creator15/2  "AmbientAirTemp"
  VI_Truck1571VinMatch/1 -> Bus Creator16/1  "F_Truck1571_VIN_Match"
  SSI2_PitchAngleExtRange/1 -> Bus Creator17/1  "PitchAngleExRange"
  Bus Creator15/1 -> Bus Creator3/13  "AMB_00"
  Bus Creator16/1 -> Bus Creator3/14  "VI_00"
  Bus Creator17/1 -> Bus Creator3/15  "SSI2_03"
  PedalPWMPos/1 -> Bus Creator8/2
  FrontAxleLeftWheelSpeed/1 -> Bus Creator18/1  "FrontAxleLeftWheelSpeed"
  FrontAxleRightWheelSpeed/1 -> Bus Creator18/2  "FrontAxleRightWheelSpeed"
  Bus Creator18/1 -> Bus Creator3/3  "HRW_0B"
  Latitude/1 -> Bus Creator19/1  "Latitude_"
  Longitude/1 -> Bus Creator19/2  "Longitude_"
  Bus Creator19/1 -> Bus Creator3/17  "PosRapidUpdate"
  HDOP/1 -> Bus Creator20/1  "HDOP_"
  Bus Creator20/1 -> Bus Creator3/18  "GNSSDOPs"
  ACCDistanceAlertSignal/1 -> Bus Creator21/1  "ACCDistanceAlertSignal"
  ForwardCollisionWarning/1 -> Bus Creator21/2  "ForwardCollisionWarning"
  Bus Creator21/1 -> Bus Creator3/9  "ACC1_2A"
  DriversDemandEngPercentTorque/1 -> Bus Creator5/4  "DriversDemandEngPercentTorque"
  PIC_Bus/1 -> Bus Creator/3
  IgnitionKeySwitch_voltage/1 -> Bus Creator8/3
  Park_brake_switch/1 -> Bus Creator9/2
  Cruise_control_enable_switch/1 -> Bus Creator9/3

== system L4_SIM/Controllers/Virtual_Controllers/L4_MABX/L4_Controller/Task_10ms ==
  In : Inport
  20msTask : Inport  Port=2
  APTC_10ms : SUB_L4_Task_10ms_SUB_APTC/APTC_10ms
  BRKPEDARB_10ms : SUB_L4_Task_10ms_SUB_BRKPEDARB/BRKPEDARB_10ms
  Bus Creator : BusCreator  Inputs=5
  FAULT_MANAGER_10ms : SUB_L4_Task_10ms_SUB_FAULT_MANAGER/FAULT_MANAGER_10ms
  STATE_CONTROL_10ms : SUB_L4_Task_10ms_SUB_STATE_CONTROL/STATE_CONTROL_10ms
  STEERCTRL_10ms : Subsystem  AncestorBlock=SUB_L4_Task_10ms_SUB_STEERCTRL/STEERCTRL_10ms
  Vehicle_speed_target : Subsystem
  10msTask : Outport
  wires:
  In/1 -> STATE_CONTROL_10ms/1, BRKPEDARB_10ms/1, STEERCTRL_10ms/2(In), APTC_10ms/1, FAULT_MANAGER_10ms/1, Vehicle_speed_target/1(In)
  APTC_10ms/1 -> Bus Creator/2  "APTC"
  Bus Creator/1 -> 10msTask/1  "10msTask"
  STEERCTRL_10ms/1(SteerCtrl_O) -> Bus Creator/1, STATE_CONTROL_10ms/3, BRKPEDARB_10ms/2  "SteeringControl"
  STATE_CONTROL_10ms/1 -> Bus Creator/3, APTC_10ms/2  "StateControl"
  BRKPEDARB_10ms/1 -> Bus Creator/4, STATE_CONTROL_10ms/2  "BrakeCtrl"
  20msTask/1 -> Vehicle_speed_target/2(20msTask), STEERCTRL_10ms/1(20msTask)
  Vehicle_speed_target/1(SpeedTarget) -> Bus Creator/5, STATE_CONTROL_10ms/4, BRKPEDARB_10ms/3

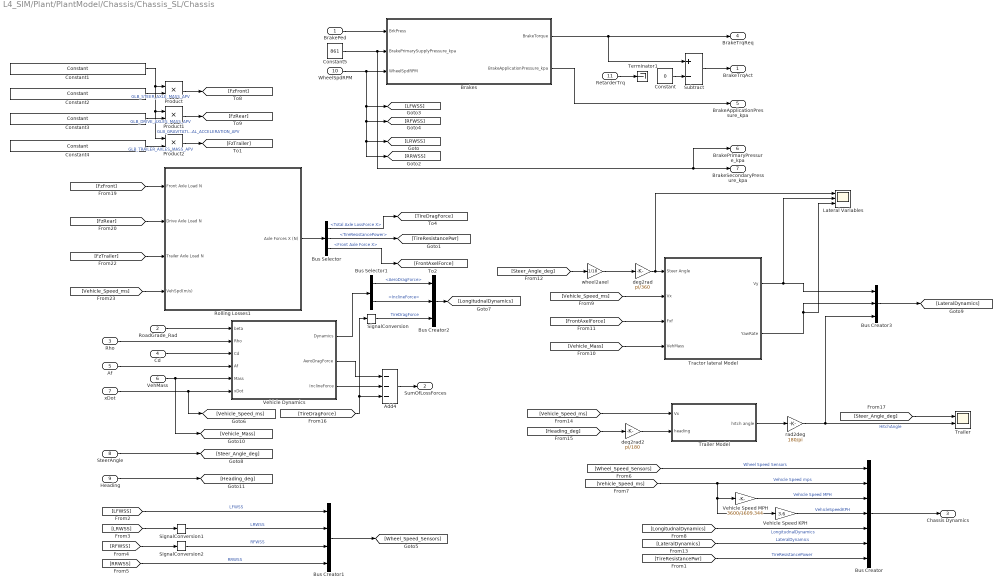
== system L4_SIM/Plant/PlantModel/Chassis/Chassis_SL/Chassis ==
  BrakePed : Inport
  RoadGrade_Rad : Inport  Port=2
  Rho : Inport  Port=3
  Cd : Inport  Port=4
  Af : Inport  Port=5
  VehMass : Inport  Port=6
  xDot : Inport  Port=7
  SteerAngle : Inport  Port=8
  Heading : Inport  Port=9
  WheelSpdRPM : Inport  Port=10
  RetarderTrq : Inport  Port=11
  Add4 : Sum  Inputs=---
  Brakes : Subsystem
  Bus Creator : BusCreator  Inputs=7
  Bus Creator1 : BusCreator  Inputs=4
  Bus Creator2 : BusCreator  Inputs=3
  Bus Creator3 : BusCreator  Inputs=3
  Bus Selector : BusSelector  OutputSignals=Total Axle LossForce X,TireResistancePower,Front Axle Force X
  Bus Selector1 : BusSelector  OutputSignals=AeroDragForce,InclineForce
  Constant : Constant  Value=0
  Constant1 : PTC_MBDS_LIB/Extras/Sources/Constant  Value2=GLB_GRAVITATIONAL_ACCELERATION_APV  PTC_MBDS_BlockVersion=5.41  PTC_BlockType=PTC_MBDS_Constant
      settings: SourceProductName=PACCAR Technical Center MBDS Library
      settings: AttributesFormatString=|
      | Value: 9.80665016174
      | Unit: 'm/s^2'
  Constant2 : PTC_MBDS_LIB/Extras/Sources/Constant  Value2=GLB_STEER_AXLE_MASS_APV  PTC_MBDS_BlockVersion=5.41  PTC_BlockType=PTC_MBDS_Constant
      settings: SourceProductName=PACCAR Technical Center MBDS Library
      settings: AttributesFormatString=|
      | Value: 5261
      | Unit: 'kg'
  Constant3 : PTC_MBDS_LIB/Extras/Sources/Constant  Value2=GLB_DRIVE_AXLES_MASS_APV  PTC_MBDS_BlockVersion=5.41  PTC_BlockType=PTC_MBDS_Constant
      settings: SourceProductName=PACCAR Technical Center MBDS Library
      settings: AttributesFormatString=|
      | Value: 11770
      | Unit: 'kg'
  Constant4 : PTC_MBDS_LIB/Extras/Sources/Constant  Value2=GLB_TRAILER_AXLES_MASS_APV  PTC_MBDS_BlockVersion=5.41  PTC_BlockType=PTC_MBDS_Constant
      settings: SourceProductName=PACCAR Technical Center MBDS Library
      settings: AttributesFormatString=|
      | Value: 12460
      | Unit: 'kg'
  Constant5 : Constant  Value=861
  Lateral Variables : Scope  NumInputPorts=3
  Product : Product  Inputs=**  OutDataTypeStr=Inherit: Inherit via back propagation  SaturateOnIntegerOverflow=on  InputSameDT=on
      settings: AttributesFormatString=Saturate: %<SaturateOnIntegerOverflow>
  Product1 : Product  Inputs=**  OutDataTypeStr=Inherit: Inherit via back propagation  SaturateOnIntegerOverflow=on  InputSameDT=on
      settings: AttributesFormatString=Saturate: %<SaturateOnIntegerOverflow>
  Product2 : Product  Inputs=**  OutDataTypeStr=Inherit: Inherit via back propagation  SaturateOnIntegerOverflow=on  InputSameDT=on
      settings: AttributesFormatString=Saturate: %<SaturateOnIntegerOverflow>
  Rolling Losses1 : Subsystem
  SignalConversion : SignalConversion  ConversionOutput=Contiguous copy  OverrideOpt=off
  SignalConversion1 : SignalConversion  ConversionOutput=Contiguous copy  OverrideOpt=off
  SignalConversion2 : SignalConversion  ConversionOutput=Contiguous copy  OverrideOpt=off
  Subtract : Sum  Inputs=+-
  Terminator1 : Terminator
  Tractor lateral Model : Subsystem
  Trailer : Scope  NumInputPorts=2
  Trailer Model : Subsystem
  Vehicle Dynamics : Subsystem
  Vehicle Speed KPH : Gain  Gain=3.6
  Vehicle Speed MPH : Gain  Gain=3600/1609.344
  deg2rad : Gain  Gain=pi/360
  "deg2rad2 " : Gain  Gain=pi/180
  rad2deg : Gain  Gain=180/pi
  wheel2axel : Gain  Gain=1/18
  BrakeTrqAct : Outport
  SumOfLossForces : Outport  Port=2
  Chassis Dynamics : Outport  Port=3
  BrakeTrqReq : Outport  Port=4
  BrakeApplicationPressure_kpa : Outport  Port=5
  BrakePrimaryPressure_kpa : Outport  Port=6
  BrakeSecondaryPressure_kpa : Outport  Port=7
  wires:
  Trailer Model/1(hitch angle) -> rad2deg/1
  rad2deg/1 -> Bus Creator3/3, Trailer/2  "HitchAngle"
  [Steer_Angle_deg] -> Trailer/1
  [Heading_deg] -> "deg2rad2 "/1
  "deg2rad2 "/1 -> Trailer Model/2(heading)
  Heading/1 -> [Heading_deg]
  [Vehicle_Speed_ms] -> Trailer Model/1(Vx)
  [Vehicle_Speed_ms] -> Tractor lateral Model/2(Vx)
  VehMass/1 -> Vehicle Dynamics/5(Mass), [Vehicle_Mass]
  [LateralDynamics] -> Bus Creator/6  "LateralDynamics"
  deg2rad/1 -> Tractor lateral Model/1(Steer Angle), Lateral Variables/1
  SteerAngle/1 -> [Steer_Angle_deg]
  [FrontAxelForce] -> Tractor lateral Model/3(Fxf)
  Bus Selector/3 -> [FrontAxelForce]  "<Front Axle Force X>"
  Bus Creator3/1 -> [LateralDynamics]
  [Vehicle_Mass] -> Tractor lateral Model/4(VehMass)
  Tractor lateral Model/2(YawRate) -> Bus Creator3/2, Lateral Variables/3
  Tractor lateral Model/1(Vy) -> Bus Creator3/1, Lateral Variables/2
  Constant5/1 -> Brakes/2(BrakePrimarySupplyPressure_kpa), BrakeSecondaryPressure_kpa/1, BrakePrimaryPressure_kpa/1
  Brakes/2(BrakeApplicationPressure_kpa) -> BrakeApplicationPressure_kpa/1
  SignalConversion2/1 -> Bus Creator1/3  "RFWSS"
  SignalConversion1/1 -> Bus Creator1/2  "LRWSS"
  SignalConversion/1 -> Bus Creator2/3  "TireDragForce"
  Constant1/1 -> Product/1, Product1/1, Product2/1  "GLB_GRAVITATIONAL_ACCELERATION_APV"
  Constant4/1 -> Product2/2  "GLB_TRAILER_AXLES_MASS_APV"
  Constant3/1 -> Product1/2  "GLB_DRIVE_AXLES_MASS_APV"
  Bus Selector1/1 -> Bus Creator2/1  "<AeroDragForce>"
  Bus Selector1/2 -> Bus Creator2/2  "<InclineForce>"
  Bus Creator2/1 -> [LongitudnalDynamics]
  Constant/1 -> Subtract/2
  Subtract/1 -> BrakeTrqAct/1
  RetarderTrq/1 -> Terminator1/1
  Bus Selector/2 -> [TireResistancePwr]  "<TireResistancePower>"
  [TireResistancePwr] -> Bus Creator/7  "TireResistancePower"
  Brakes/1(BrakeTorque) -> Subtract/1, BrakeTrqReq/1
  WheelSpdRPM/1 -> Brakes/3(WheelSpdRPM), [RRWSS], [LRWSS], [RFWSS], [LFWSS]
  BrakePed/1 -> Brakes/1(BrkPress)
  Add4/1 -> SumOfLossForces/1
  Vehicle Dynamics/2(AeroDragForce) -> Add4/1
  Vehicle Dynamics/3(InclineForce) -> Add4/2
  [TireDragForce] -> Add4/3, SignalConversion/1
  xDot/1 -> [Vehicle_Speed_ms], Vehicle Dynamics/6(xDot)
  Af/1 -> Vehicle Dynamics/4(Af)
  Cd/1 -> Vehicle Dynamics/3(Cd)
  Rho/1 -> Vehicle Dynamics/2(Rho)
  Vehicle Speed MPH/1 -> Bus Creator/3  "Vehicle Speed MPH"
  [Vehicle_Speed_ms] -> Bus Creator/2, Vehicle Speed MPH/1, Vehicle Speed KPH/1  "Vehicle Speed mps"
  Bus Creator/1 -> Chassis Dynamics/1
  [Wheel_Speed_Sensors] -> Bus Creator/1  "Wheel Speed Sensors"
  [RRWSS] -> Bus Creator1/4  "RRWSS"
  [LRWSS] -> SignalConversion1/1
  [RFWSS] -> SignalConversion2/1
  [LFWSS] -> Bus Creator1/1  "LFWSS"
  Bus Creator1/1 -> [Wheel_Speed_Sensors]
  RoadGrade_Rad/1 -> Vehicle Dynamics/1(beta)
  Vehicle Speed KPH/1 -> Bus Creator/4  "VehicleSpeedKPH"
  [FzTrailer] -> Rolling Losses1/3(Trailer Axle Load N)
  [FzRear] -> Rolling Losses1/2(Drive Axle Load N)
  [FzFront] -> Rolling Losses1/1(Front Axle Load N)
  [Vehicle_Speed_ms] -> Rolling Losses1/4(VehSpd(m/s))
  Rolling Losses1/1("Axle Forces X (N) ") -> Bus Selector/1
  Bus Selector/1 -> [TireDragForce]  "<Total Axle LossForce X>"
  Product/1 -> [FzFront]
  Product1/1 -> [FzRear]
  Constant2/1 -> Product/2  "GLB_STEER_AXLE_MASS_APV"
  Product2/1 -> [FzTrailer]
  Vehicle Dynamics/1(Dynamics) -> Bus Selector1/1
  [LongitudnalDynamics] -> Bus Creator/5  "LongitudnalDynamics"
  [Steer_Angle_deg] -> wheel2axel/1
  wheel2axel/1 -> deg2rad/1

== system L4_SIM/Plant/PlantModel/Chassis/Chassis_SL/DriveAxleLosses ==
  AxleTrq : Inport
  AxleRPM : Inport  Port=2
  AxleEff : Inport  Port=3
  2D_Lookup_Table : PTC_MBDS_LIB/Extras/Lookup Tables/2D_Lookup_Table  ParameterObjectName=GLB_AXLE_POWER_LOSS_DATA_MPV  InterpolationMethod=Linear  PTC_MBDS_BlockVersion=5.41  PTC_BlockType=PTC_MBDS_2D_Lookup_Table
      settings: SourceProductName=PACCAR Technical Center MBDS Library
      settings: AttributesFormatString=|
      | Row Axis: GLB_AXLE_POWER_LOSS_AXLETRQ_STEP_MPV (N*m)
      | Column Axis: GLB_AXLE_POWER_LOSS_AXLESPD_STEP_MPV (rpm)
      | Data Axis: GLB_AXLE_POWER_LOSS_DATA_MPV (kW)
      | Interpolation Method: Linear
  2D_Lookup_Table1 : PTC_MBDS_LIB/Extras/Lookup Tables/2D_Lookup_Table  ParameterObjectName=GLB_AXLE_POWER_LOSS_DATA_MPV  InterpolationMethod=Linear  PTC_MBDS_BlockVersion=5.41  PTC_BlockType=PTC_MBDS_2D_Lookup_Table
      settings: SourceProductName=PACCAR Technical Center MBDS Library
      settings: AttributesFormatString=|
      | Row Axis: GLB_AXLE_POWER_LOSS_AXLETRQ_STEP_MPV (N*m)
      | Column Axis: GLB_AXLE_POWER_LOSS_AXLESPD_STEP_MPV (rpm)
      | Data Axis: GLB_AXLE_POWER_LOSS_DATA_MPV (kW)
      | Interpolation Method: Linear
  Add : Sum
  Add1 : Sum
  Add2 : Sum  Inputs=-+
  Add3 : Sum
  AxlePowerSplit : Gain  Gain=0.7
  AxlePowerSplit1 : Gain  Gain=1-0.7
  BearingLossesNm : Constant  Value=1.8
  Compare To Zero : simulink/Logic and Bit Operations/Compare To Zero  relop=>  OutDataTypeStr=boolean
  Divide_gtz : Subsystem
  Product : Product  Inputs=**
  Product1 : Product  Inputs=**
  Product2 : Product  Inputs=**
  RPM2RADS : Gain  Gain=pi/30
  Saturation : Saturate  UpperLimit=Inf  LowerLimit=0
  W2kW : Gain  Gain=1/1000
  W2kW1 : Gain  Gain=1/1000
  kW2W : Gain  Gain=1000
  o : Constant
  AxleLossTorque : Outport
  AxleLossPower : Outport  Port=2
  wires:
  Divide_gtz/1(out) -> AxleLossTorque/1
  Add3/1 -> Add1/2
  AxlePowerSplit1/1 -> Product2/1, 2D_Lookup_Table1/1
  AxlePowerSplit/1 -> 2D_Lookup_Table/1
  2D_Lookup_Table1/1 -> Add3/2
  2D_Lookup_Table/1 -> Add3/1
  Product2/1 -> W2kW1/1
  W2kW1/1 -> Product1/2
  Compare To Zero/1 -> Divide_gtz/Enable
  o/1 -> Add2/2
  Product1/1 -> Add1/1
  AxleEff/1 -> Add2/1
  Add2/1 -> Product1/1
  RPM2RADS/1 -> Divide_gtz/2(den), Compare To Zero/1, Product/2, Product2/2
  W2kW/1 -> Add/2
  Add/1 -> kW2W/1
  Product/1 -> W2kW/1
  BearingLossesNm/1 -> Product/1
  Add1/1 -> Saturation/1
  AxleTrq/1 -> AxlePowerSplit1/1, AxlePowerSplit/1
  kW2W/1 -> Divide_gtz/1(num), AxleLossPower/1
  Saturation/1 -> Add/1
  AxleRPM/1 -> RPM2RADS/1, 2D_Lookup_Table1/2, 2D_Lookup_Table/2
